simulink model "ex0"  (R2025a)
settings: Solver=VariableStepAuto  StartTime=0.0  StopTime=10.0  RelTol=1e-3
settings Model: Creator=sphuwaset_ros  LastModifiedBy=sphuwaset_ros

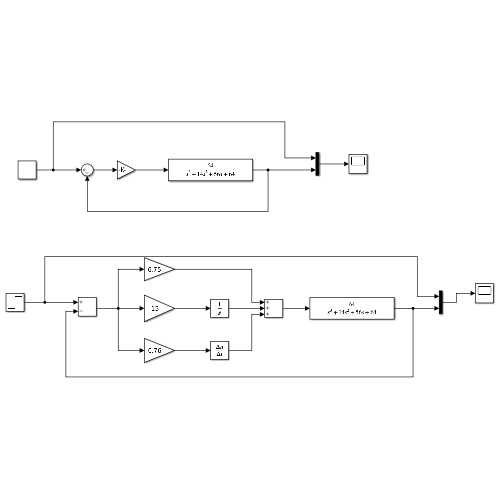
[thumbnail: Simulink's stored preview of the top-level diagram]
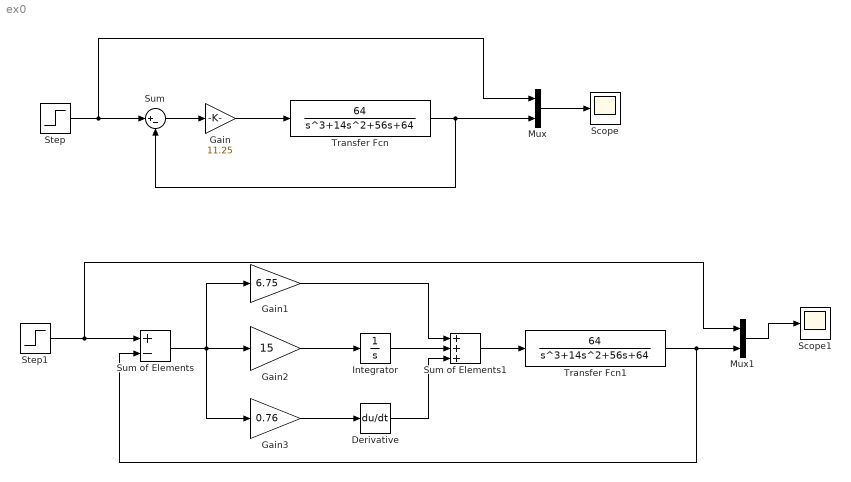
== system ex0 ==
  Derivative : Derivative
  Gain : Gain  Gain=11.25
  Gain1 : Gain  Gain=6.75
  Gain2 : Gain  Gain=15
  Gain3 : Gain  Gain=0.76
  Integrator : Integrator
  Mux : Mux  Inputs=2
  Mux1 : Mux  Inputs=2
  Scope : Scope
      settings: ActiveDisplayYMinimum=-0.96077114769417937  ActiveDisplayYMaximum=5.5579057676408956
  Scope1 : Scope
      settings: ActiveDisplayYMinimum=-1.1010303332679374  ActiveDisplayYMaximum=3.5316716476109082
  Step : Step  SampleTime=0  ZeroCross=off
  Step1 : Step  SampleTime=0
  Sum : Sum  Inputs=|+-
  Sum of Elements : Sum  Inputs=+-
  Sum of Elements1 : Sum  Inputs=+++
  Transfer Fcn : TransferFcn  Numerator=[64]  Denominator=[1 14 56 64]
  Transfer Fcn1 : TransferFcn  Numerator=[64]  Denominator=[1 14 56 64]
  wires:
  Gain/1 -> Transfer Fcn/1
  Transfer Fcn/1 -> Sum/2, Mux/2
  Sum/1 -> Gain/1
  Step/1 -> Sum/1, Mux/1
  Mux/1 -> Scope/1
  Step1/1 -> Mux1/1, Sum of Elements/1
  Sum of Elements/1 -> Gain3/1, Gain1/1, Gain2/1
  Gain2/1 -> Integrator/1
  Gain1/1 -> Sum of Elements1/1
  Integrator/1 -> Sum of Elements1/2
  Gain3/1 -> Derivative/1
  Derivative/1 -> Sum of Elements1/3
  Sum of Elements1/1 -> Transfer Fcn1/1
  Transfer Fcn1/1 -> Mux1/2, Sum of Elements/2
  Mux1/1 -> Scope1/1
